simulink model "ABS_virtual_no_fliter_40_88"  (R2023a)
settings: Solver=VariableStepAuto  StartTime=0.0  StopTime=inf  FixedStep=0.001  RelTol=1e-3  EnableMultiTasking=on
PreLoadFcn:
  | SoftABS_params
libraries: CarMaker4SL x28, simulink x19, dspsigops x5
(part 2 of 3)

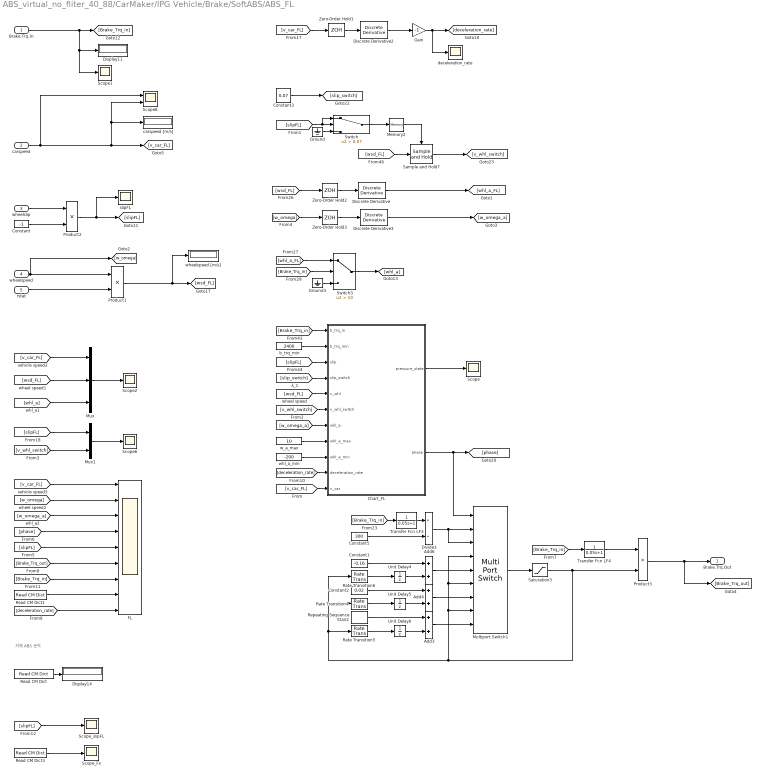
== system ABS_virtual_no_fliter_40_88/CarMaker/IPG Vehicle/Brake/SoftABS/ABS_FL ==
  note: 자체 ABS 로직
  Brake.Trq.In : Inport
  carspeed : Inport  Port=2
  wheelslip : Inport  Port=3
  wheelspeed : Inport  Port=4
  rstat : Inport  Port=5
  Add3 : Sum
  Add4 : Sum
  Add6 : Sum
  Chart_FL : Stateflow chart  TreatAsAtomicUnit=on
      settings: PortSchema="{\"entries\":[{\"content\":{\"sides\":[{\"content\":{\"connectorIds\":[\"In1\",\"In3\",\"In2\",\"In4\",\"In5\",\"In6\",\"In7\",\"In8\",\"In9\",\"In10\",\"In11\"]},\"type\":\"ConnectorPlacement.EquallySpacedRectSide\",\"uuid\":\"cdedcea2-93f8-4775-9e06-e6ef8db0f566\"},{\"content\":{\"connectorIds\":[\"Out1\",\"Out2\"],\"side\":\"RIGHT\"},\"type\":\"ConnectorPlacement.EquallySpacedRectSide\",\"uuid\":\"86cd5634-3296-4603-b9fe-1da91bf44691\"},{\"content\":{\"side\":\"TOP\"},\"type\":\"ConnectorPlacement.EquallySpacedRectSide\",\"uuid\":\"3d39226d-e82c-42be-bb61-abed7a445d69\"}]},\"type\":\"ConnectorPlacement.EquallySpacedConnector\",\"uuid\":\"e0869cc4-498e-4360-9359-f4884b7944df\"}],\"packageUris\":[\"http://schema.mathworks.com/mf0/Connector/R2020b\"],\"version\":\"1.0\"}"
  Constant : Constant  Value=-1
  Constant1 : Constant  Value=-0.16
  Constant2 : Constant  Value=0.02
  Constant3 : Constant  Value=0.07
  Constant5 : Constant  Value=300
  Discrete Derivative : simulink/Discrete/Discrete Derivative  gainval=1.0  ICPrevScaledInput=0.0  OutMin=[]  OutMax=[]  OutDataType=fixdt(1, 16)  OutScaling=2^-10  DoSatur=off
  Discrete Derivative2 : simulink/Discrete/Discrete Derivative  gainval=1.0  ICPrevScaledInput=0.0  OutMin=[]  OutMax=[]  OutDataType=fixdt(1, 16)  OutScaling=2^-10  DoSatur=off
  Discrete Derivative3 : simulink/Discrete/Discrete Derivative  gainval=1.0  ICPrevScaledInput=0.0  OutMin=[]  OutMax=[]  OutDataType=fixdt(1, 16)  OutScaling=2^-10  DoSatur=off
  Display11 : Display
  Display14 : Display
  Divide3 : Product  Inputs=*/
  FL : Scope  NumInputPorts=9
  Gain : Gain  Gain=-1
  Ground : Ground
  Ground3 : Ground
  Memory2 : Memory  InheritSampleTime=on
  Multiport Switch1 : MultiPortSwitch  DataPortOrder=Zero-based contiguous  Inputs=8  zeroidx=on  SaturateOnIntegerOverflow=off  InputSameDT=off
  Mux : Mux  Inputs=3
  Mux1 : Mux  Inputs=2
  Product1 : Product
  Product2 : Product
  Product3 : Product  InputSameDT=on  SaturateOnIntegerOverflow=on  OutDataTypeStr=Inherit: Same as first input
  Rate Transition4 : RateTransition  OutPortSampleTime=0.001
  Rate Transition5 : RateTransition  OutPortSampleTime=0.001
  Rate Transition6 : RateTransition  OutPortSampleTime=0.001
  Read CM Dict : CarMaker4SL/Read CM Dict  xname=DM.Long.StepDist  xsync=off  xstime=Continuous
  Read CM Dict1 : CarMaker4SL/Read CM Dict  xname=Car.FxFL  xsync=off  xstime=Continuous
  Read CM Dict3 : CarMaker4SL/Read CM Dict  xname=Car.FxFL  xsync=off  xstime=Continuous
  Repeating Sequence Stair2 : simulink/Sources/Repeating Sequence Stair  OutValues=[0.02 0].'  tsamp=0.001  OutMin=[]  OutMax=[]  OutDataTypeStr=double  OutputDataTypeScalingMode=double  OutDataType=fixdt(0,8)  ConRadixGroup=Best Precision: Vector-wise  OutScaling=2^-12
  Sample and Hold7 : dspsigops/Sample and Hold  trig=Rising edge  initCond=0  latchinput=off
  Saturation3 : Saturate  UpperLimit=1  LowerLimit=0
  Scope{,1..2,6} (4 alike) : Scope
  Scope8 : Scope  NumInputPorts=2
  Scope_Fx : Scope
  Scope_slipFL : Scope
  Switch : Switch  Criteria=u2 > Threshold  Threshold=0.07  SaturateOnIntegerOverflow=off  InputSameDT=off
  Switch3 : Switch  Criteria=u2 > Threshold  Threshold=10  SaturateOnIntegerOverflow=off  InputSameDT=off
  Transfer Fcn LF3 : TransferFcn  Denominator=[0.05 1]
  Transfer Fcn LF4 : TransferFcn  Denominator=[0.05 1]
  Unit Delay4 : UnitDelay  SampleTime=0.001  HasFrameUpgradeWarning=on
  Unit Delay5 : UnitDelay  SampleTime=0.001  HasFrameUpgradeWarning=on
  Unit Delay6 : UnitDelay  SampleTime=0.001  HasFrameUpgradeWarning=on
  Zero-Order Hold1 : ZeroOrderHold  SampleTime=0.001
  Zero-Order Hold2 : ZeroOrderHold  SampleTime=0.001
  Zero-Order Hold3 : ZeroOrderHold  SampleTime=0.001
  b_trq_min : Constant  Value=2400
  carspeed [m/s] : Display
  deceleration_rate : Scope
  slipFL : Scope
  w_a_max : Constant  Value=10
  wheelspeed [m/s] : Display
  whl_a_min : Constant  Value=-200
  Brake.Trq.Out : Outport  VectorParamsAs1DForOutWhenUnconnected=off
  wires:
  [wsd_FL] -> Zero-Order Hold2/1
  rstat/1 -> Product1/2
  Brake.Trq.In/1 -> Scope1/1, Display11/1, [Brake_Trq_in]
  Read CM Dict/1 -> Display14/1
  wheelslip/1 -> Product2/1
  Product2/1 -> slipFL/1, [slipFL]
  Constant/1 -> Product2/2
  carspeed/1 -> [v_car_FL], Scope8/2, carspeed [m/s]/1, Scope8/1
  [Brake_Trq_in] -> Switch3/2
  Ground3/1 -> Switch3/3
  Switch3/1 -> [whl_a]
  [whl_a_FL] -> Switch3/1
  [Brake_Trq_in] -> Chart_FL/1(b_trq_in)
  b_trq_min/1 -> Chart_FL/3(b_trq_min)
  [slipFL] -> Chart_FL/2(slip)
  Chart_FL/2(phase) -> [phase], Multiport Switch1/1
  Chart_FL/1(pressure_state) -> Scope/1
  [slipFL] -> Switch/1, Switch/2
  Constant3/1 -> [slip_switch]
  Switch/1 -> Memory2/1
  [wsd_FL] -> Sample and Hold7/1
  Sample and Hold7/1 -> [v_whl_switch]
  [slip_switch] -> Chart_FL/4(slip_switch)
  [w_omega_a] -> Chart_FL/7(whl_a)
  whl_a_min/1 -> Chart_FL/9(whl_a_min)
  w_a_max/1 -> Chart_FL/8(whl_a_max)
  [wsd_FL] -> Chart_FL/5(v_whl)
  Ground/1 -> Switch/3
  Memory2/1 -> Sample and Hold7/Trigger
  [v_car_FL] -> Mux/1
  [wsd_FL] -> Mux/2
  [whl_a] -> Mux/3
  Mux/1 -> Scope2/1
  [slipFL] -> Mux1/1
  [v_whl_switch] -> Mux1/2
  Mux1/1 -> Scope6/1
  [w_omega] -> FL/2
  [v_car_FL] -> FL/1
  [w_omega_a] -> FL/3
  [phase] -> FL/4
  [slipFL] -> FL/5
  [Brake_Trq_out] -> FL/6
  [Brake_Trq_in] -> FL/7
  Read CM Dict1/1 -> FL/8
  Discrete Derivative2/1 -> Gain/1
  Gain/1 -> deceleration_rate/1, [deceleration_rate]
  [v_car_FL] -> Chart_FL/11(v_car)
  [v_car_FL] -> Zero-Order Hold1/1
  [v_whl_switch] -> Chart_FL/6(v_whl_switch)
  [w_omega] -> Zero-Order Hold3/1
  wheelspeed/1 -> [w_omega], Product1/1
  Discrete Derivative/1 -> [whl_a_FL]
  Product1/1 -> [wsd_FL], wheelspeed [m/s]/1
  Zero-Order Hold1/1 -> Discrete Derivative2/1
  Zero-Order Hold2/1 -> Discrete Derivative/1
  Zero-Order Hold3/1 -> Discrete Derivative3/1
  Rate Transition4/1 -> Unit Delay5/1
  Unit Delay5/1 -> Add4/2
  Add4/1 -> Multiport Switch1/7
  Transfer Fcn LF4/1 -> Product3/1
  Repeating Sequence Stair2/1 -> Add3/1
  [Brake_Trq_in] -> Transfer Fcn LF3/1
  Add3/1 -> Multiport Switch1/9
  Saturation3/1 -> Multiport Switch1/8, Multiport Switch1/6, Multiport Switch1/4, Rate Transition5/1, Rate Transition4/1, Rate Transition6/1, Product3/2
  Multiport Switch1/1 -> Saturation3/1
  [Brake_Trq_in] -> Transfer Fcn LF4/1
  Divide3/1 -> Multiport Switch1/3, Multiport Switch1/2
  Product3/1 -> Brake.Trq.Out/1, [Brake_Trq_out]
  Unit Delay4/1 -> Add6/2
  Constant2/1 -> Add4/1
  Transfer Fcn LF3/1 -> Divide3/1
  Rate Transition5/1 -> Unit Delay6/1
  Constant1/1 -> Add6/1
  Unit Delay6/1 -> Add3/2
  Rate Transition6/1 -> Unit Delay4/1
  Constant5/1 -> Divide3/2
  Add6/1 -> Multiport Switch1/5
  Discrete Derivative3/1 -> [w_omega_a]
  [deceleration_rate] -> FL/9
  [deceleration_rate] -> Chart_FL/10(deceleration_rate)
  Read CM Dict3/1 -> Scope_Fx/1
  [slipFL] -> Scope_slipFL/1

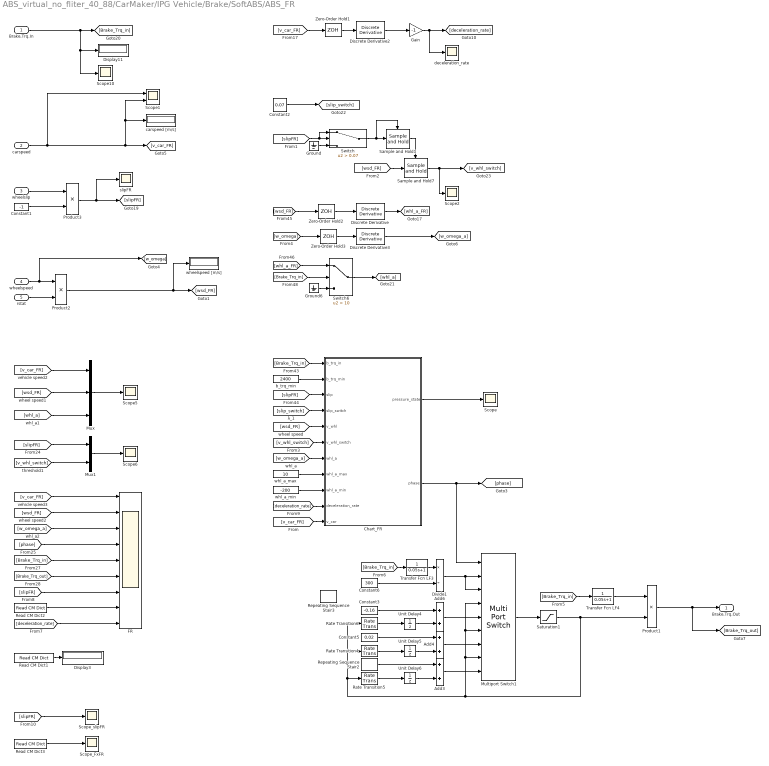
== system ABS_virtual_no_fliter_40_88/CarMaker/IPG Vehicle/Brake/SoftABS/ABS_FR ==
  Brake.Trq.In : Inport
  carspeed : Inport  Port=2
  wheelslip : Inport  Port=3
  wheelspeed : Inport  Port=4
  rstat : Inport  Port=5
  Add3 : Sum
  Add4 : Sum
  Add6 : Sum
  Chart_FR : Stateflow chart  TreatAsAtomicUnit=on
      settings: PortSchema="{\"entries\":[{\"content\":{\"sides\":[{\"content\":{\"connectorIds\":[\"In1\",\"In3\",\"In2\",\"In4\",\"In5\",\"In6\",\"In7\",\"In8\",\"In9\",\"In10\",\"In11\"]},\"type\":\"ConnectorPlacement.EquallySpacedRectSide\",\"uuid\":\"cdedcea2-93f8-4775-9e06-e6ef8db0f566\"},{\"content\":{\"connectorIds\":[\"Out1\",\"Out2\"],\"side\":\"RIGHT\"},\"type\":\"ConnectorPlacement.EquallySpacedRectSide\",\"uuid\":\"86cd5634-3296-4603-b9fe-1da91bf44691\"},{\"content\":{\"side\":\"TOP\"},\"type\":\"ConnectorPlacement.EquallySpacedRectSide\",\"uuid\":\"3d39226d-e82c-42be-bb61-abed7a445d69\"}]},\"type\":\"ConnectorPlacement.EquallySpacedConnector\",\"uuid\":\"e0869cc4-498e-4360-9359-f4884b7944df\"}],\"packageUris\":[\"http://schema.mathworks.com/mf0/Connector/R2020b\"],\"version\":\"1.0\"}"
  Constant1 : Constant  Value=-1
  Constant2 : Constant  Value=0.07
  Constant3 : Constant  Value=-0.16
  Constant5 : Constant  Value=0.02
  Constant6 : Constant  Value=300
  Discrete Derivative : simulink/Discrete/Discrete Derivative  gainval=1.0  ICPrevScaledInput=0.0  OutMin=[]  OutMax=[]  OutDataType=fixdt(1, 16)  OutScaling=2^-10  DoSatur=off
  Discrete Derivative2 : simulink/Discrete/Discrete Derivative  gainval=1.0  ICPrevScaledInput=0.0  OutMin=[]  OutMax=[]  OutDataType=fixdt(1, 16)  OutScaling=2^-10  DoSatur=off
  Discrete Derivative3 : simulink/Discrete/Discrete Derivative  gainval=1.0  ICPrevScaledInput=0.0  OutMin=[]  OutMax=[]  OutDataType=fixdt(1, 16)  OutScaling=2^-10  DoSatur=off
  Display11 : Display
  Display3 : Display
  Divide1 : Product  Inputs=*/
  FR : Scope  NumInputPorts=9
  Gain : Gain  Gain=-1
  Ground : Ground
  Ground6 : Ground
  Multiport Switch1 : MultiPortSwitch  DataPortOrder=Zero-based contiguous  Inputs=8  zeroidx=on  SaturateOnIntegerOverflow=off  InputSameDT=off
  Mux : Mux  Inputs=3
  Mux1 : Mux  Inputs=2
  Product1 : Product  InputSameDT=on  SaturateOnIntegerOverflow=on  OutDataTypeStr=Inherit: Same as first input
  Product2 : Product
  Product3 : Product
  Rate Transition4 : RateTransition  OutPortSampleTime=0.001
  Rate Transition5 : RateTransition  OutPortSampleTime=0.001
  Rate Transition6 : RateTransition  OutPortSampleTime=0.001
  Read CM Dict1 : CarMaker4SL/Read CM Dict  xname=DM.Long.StepDist  xsync=off  xstime=Continuous
  Read CM Dict2 : CarMaker4SL/Read CM Dict  xname=Car.FxFR  xsync=off  xstime=Continuous
  Read CM Dict3 : CarMaker4SL/Read CM Dict  xname=Car.FxFR  xsync=off  xstime=Continuous
  Repeating Sequence Stair2 : simulink/Sources/Repeating Sequence Stair  OutValues=[0.02 0].'  tsamp=0.001  OutMin=[]  OutMax=[]  OutDataTypeStr=double  OutputDataTypeScalingMode=double  OutDataType=fixdt(0,8)  ConRadixGroup=Best Precision: Vector-wise  OutScaling=2^-12
  Repeating Sequence Stair3 : simulink/Sources/Repeating Sequence Stair  OutValues=[-0.16 0].'  tsamp=0.001  OutMin=[]  OutMax=[]  OutDataTypeStr=double  OutputDataTypeScalingMode=double  OutDataType=fixdt(0,8)  ConRadixGroup=Best Precision: Vector-wise  OutScaling=2^-12
  Sample and Hold1 : dspsigops/Sample and Hold  trig=Rising edge  initCond=0  latchinput=off
  Sample and Hold7 : dspsigops/Sample and Hold  trig=Rising edge  initCond=0  latchinput=off
  Saturation1 : Saturate  UpperLimit=1  LowerLimit=0
  Scope{,2,5..6,10} (5 alike) : Scope
  Scope1 : Scope  NumInputPorts=2
  Scope_FxFR : Scope
  Scope_slipFR : Scope
  Switch : Switch  Criteria=u2 > Threshold  Threshold=0.07  SaturateOnIntegerOverflow=off  InputSameDT=off
  Switch6 : Switch  Criteria=u2 > Threshold  Threshold=10  SaturateOnIntegerOverflow=off  InputSameDT=off
  Transfer Fcn LF3 : TransferFcn  Denominator=[0.05 1]
  Transfer Fcn LF4 : TransferFcn  Denominator=[0.05 1]
  Unit Delay4 : UnitDelay  SampleTime=0.001  HasFrameUpgradeWarning=on
  Unit Delay5 : UnitDelay  SampleTime=0.001  HasFrameUpgradeWarning=on
  Unit Delay6 : UnitDelay  SampleTime=0.001  HasFrameUpgradeWarning=on
  Zero-Order Hold1 : ZeroOrderHold  SampleTime=0.001
  Zero-Order Hold2 : ZeroOrderHold  SampleTime=0.001
  Zero-Order Hold3 : ZeroOrderHold  SampleTime=0.001
  b_trq_min : Constant  Value=2400
  carspeed [m/s] : Display
  deceleration_rate : Scope
  slipFR : Scope
  wheelspeed [m/s] : Display
  whl_a_max : Constant  Value=10
  whl_a_min : Constant  Value=-200
  Brake.Trq.Out : Outport  VectorParamsAs1DForOutWhenUnconnected=off
  wires:
  Switch6/1 -> [whl_a]
  Read CM Dict1/1 -> Display3/1
  Ground6/1 -> Switch6/3
  [Brake_Trq_in] -> Switch6/2
  [whl_a_FR] -> Switch6/1
  wheelslip/1 -> Product3/1
  Constant1/1 -> Product3/2
  Product3/1 -> slipFR/1, [slipFR]
  rstat/1 -> Product2/2
  Discrete Derivative/1 -> [whl_a_FR]
  Brake.Trq.In/1 -> Scope10/1, Display11/1, [Brake_Trq_in]
  [wsd_FR] -> Zero-Order Hold2/1
  carspeed/1 -> Scope1/2, carspeed [m/s]/1, [v_car_FR], Scope1/1
  Constant2/1 -> [slip_switch]
  Chart_FR/1(pressure_state) -> Scope/1
  Chart_FR/2(phase) -> [phase], Multiport Switch1/1
  [whl_a] -> Mux/3
  [slipFR] -> FR/7
  [wsd_FR] -> Mux/2
  Mux/1 -> Scope5/1
  [v_whl_switch] -> Mux1/2
  [slipFR] -> Mux1/1
  [v_car_FR] -> FR/1
  [Brake_Trq_in] -> FR/5
  [w_omega_a] -> FR/3
  [Brake_Trq_out] -> FR/6
  [v_car_FR] -> Mux/1
  [phase] -> FR/4
  [wsd_FR] -> FR/2
  Mux1/1 -> Scope6/1
  Read CM Dict2/1 -> FR/8
  Product2/1 -> [wsd_FR], wheelspeed [m/s]/1
  Discrete Derivative2/1 -> Gain/1
  [v_car_FR] -> Zero-Order Hold1/1
  Gain/1 -> deceleration_rate/1, [deceleration_rate]
  [v_whl_switch] -> Chart_FR/6(v_whl_switch)
  b_trq_min/1 -> Chart_FR/3(b_trq_min)
  [v_car_FR] -> Chart_FR/11(v_car)
  whl_a_max/1 -> Chart_FR/8(whl_a_max)
  [w_omega_a] -> Chart_FR/7(whl_a)
  [slipFR] -> Chart_FR/2(slip)
  [wsd_FR] -> Chart_FR/5(v_whl)
  [Brake_Trq_in] -> Chart_FR/1(b_trq_in)
  whl_a_min/1 -> Chart_FR/9(whl_a_min)
  [slip_switch] -> Chart_FR/4(slip_switch)
  Switch/1 -> Sample and Hold1/1, Sample and Hold1/Trigger
  Ground/1 -> Switch/3
  [wsd_FR] -> Sample and Hold7/1
  [slipFR] -> Switch/1, Switch/2
  Sample and Hold7/1 -> Scope2/1, [v_whl_switch]
  [w_omega] -> Zero-Order Hold3/1
  wheelspeed/1 -> [w_omega], Product2/1
  Sample and Hold1/1 -> Sample and Hold7/Trigger
  Zero-Order Hold1/1 -> Discrete Derivative2/1
  Zero-Order Hold2/1 -> Discrete Derivative/1
  Zero-Order Hold3/1 -> Discrete Derivative3/1
  Rate Transition4/1 -> Unit Delay5/1
  Unit Delay5/1 -> Add4/2
  Add4/1 -> Multiport Switch1/7
  Transfer Fcn LF4/1 -> Product1/1
  Repeating Sequence Stair2/1 -> Add3/1
  [Brake_Trq_in] -> Transfer Fcn LF3/1
  Add3/1 -> Multiport Switch1/9
  Saturation1/1 -> Multiport Switch1/8, Multiport Switch1/6, Multiport Switch1/4, Rate Transition6/1, Rate Transition4/1, Rate Transition5/1, Product1/2
  Multiport Switch1/1 -> Saturation1/1
  [Brake_Trq_in] -> Transfer Fcn LF4/1
  Divide1/1 -> Multiport Switch1/3, Multiport Switch1/2
  Product1/1 -> Brake.Trq.Out/1, [Brake_Trq_out]
  Unit Delay4/1 -> Add6/2
  Constant5/1 -> Add4/1
  Transfer Fcn LF3/1 -> Divide1/1
  Rate Transition5/1 -> Unit Delay6/1
  Constant3/1 -> Add6/1
  Unit Delay6/1 -> Add3/2
  Rate Transition6/1 -> Unit Delay4/1
  Constant6/1 -> Divide1/2
  Add6/1 -> Multiport Switch1/5
  Discrete Derivative3/1 -> [w_omega_a]
  [deceleration_rate] -> FR/9
  [deceleration_rate] -> Chart_FR/10(deceleration_rate)
  Read CM Dict3/1 -> Scope_FxFR/1
  [slipFR] -> Scope_slipFR/1

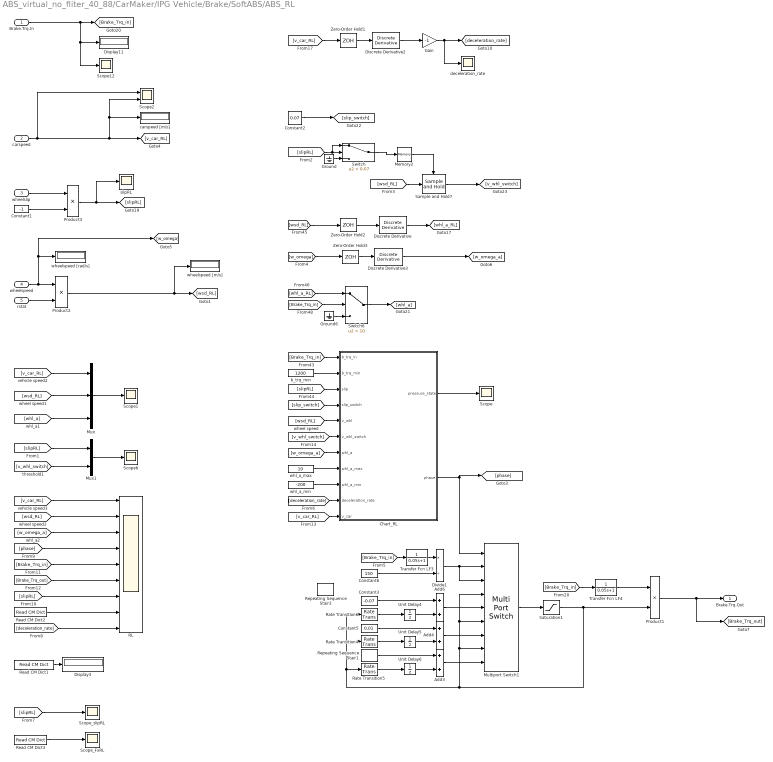
== system ABS_virtual_no_fliter_40_88/CarMaker/IPG Vehicle/Brake/SoftABS/ABS_RL ==
  Brake.Trq.In : Inport
  carspeed : Inport  Port=2
  wheelslip : Inport  Port=3
  wheelspeed : Inport  Port=4
  rstat : Inport  Port=5
  Add3 : Sum
  Add4 : Sum
  Add6 : Sum
  Chart_RL : Stateflow chart  TreatAsAtomicUnit=on
      settings: PortSchema="{\"entries\":[{\"content\":{\"sides\":[{\"content\":{\"connectorIds\":[\"In1\",\"In3\",\"In2\",\"In4\",\"In5\",\"In6\",\"In7\",\"In8\",\"In9\",\"In10\",\"In11\"]},\"type\":\"ConnectorPlacement.EquallySpacedRectSide\",\"uuid\":\"cdedcea2-93f8-4775-9e06-e6ef8db0f566\"},{\"content\":{\"connectorIds\":[\"Out1\",\"Out2\"],\"side\":\"RIGHT\"},\"type\":\"ConnectorPlacement.EquallySpacedRectSide\",\"uuid\":\"86cd5634-3296-4603-b9fe-1da91bf44691\"},{\"content\":{\"side\":\"TOP\"},\"type\":\"ConnectorPlacement.EquallySpacedRectSide\",\"uuid\":\"3d39226d-e82c-42be-bb61-abed7a445d69\"}]},\"type\":\"ConnectorPlacement.EquallySpacedConnector\",\"uuid\":\"e0869cc4-498e-4360-9359-f4884b7944df\"}],\"packageUris\":[\"http://schema.mathworks.com/mf0/Connector/R2020b\"],\"version\":\"1.0\"}"
  Constant1 : Constant  Value=-1
  Constant2 : Constant  Value=0.07
  Constant3 : Constant  Value=-0.07
  Constant5 : Constant  Value=0.01
  Constant6 : Constant  Value=150
  Discrete Derivative : simulink/Discrete/Discrete Derivative  gainval=1.0  ICPrevScaledInput=0.0  OutMin=[]  OutMax=[]  OutDataType=fixdt(1, 16)  OutScaling=2^-10  DoSatur=off
  Discrete Derivative2 : simulink/Discrete/Discrete Derivative  gainval=1.0  ICPrevScaledInput=0.0  OutMin=[]  OutMax=[]  OutDataType=fixdt(1, 16)  OutScaling=2^-10  DoSatur=off
  Discrete Derivative3 : simulink/Discrete/Discrete Derivative  gainval=1.0  ICPrevScaledInput=0.0  OutMin=[]  OutMax=[]  OutDataType=fixdt(1, 16)  OutScaling=2^-10  DoSatur=off
  Display11 : Display
  Display3 : Display
  Divide1 : Product  Inputs=*/
  Gain : Gain  Gain=-1
  Ground : Ground
  Ground6 : Ground
  Memory2 : Memory  InheritSampleTime=on
  Multiport Switch1 : MultiPortSwitch  DataPortOrder=Zero-based contiguous  Inputs=8  zeroidx=on  SaturateOnIntegerOverflow=off  InputSameDT=off
  Mux : Mux  Inputs=3
  Mux1 : Mux  Inputs=2
  Product1 : Product  InputSameDT=on  SaturateOnIntegerOverflow=on  OutDataTypeStr=Inherit: Same as first input
  Product2 : Product
  Product3 : Product
  RL : Scope  NumInputPorts=9
  Rate Transition4 : RateTransition  OutPortSampleTime=0.001
  Rate Transition5 : RateTransition  OutPortSampleTime=0.001
  Rate Transition6 : RateTransition  OutPortSampleTime=0.001
  Read CM Dict1 : CarMaker4SL/Read CM Dict  xname=DM.Long.StepDist  xsync=off  xstime=Continuous
  Read CM Dict2 : CarMaker4SL/Read CM Dict  xname=Car.FxRL  xsync=off  xstime=Continuous
  Read CM Dict3 : CarMaker4SL/Read CM Dict  xname=Car.FxRL  xsync=off  xstime=Continuous
  Repeating Sequence Stair1 : simulink/Sources/Repeating Sequence Stair  OutValues=[0.07 0].'  tsamp=0.001  OutMin=[]  OutMax=[]  OutDataTypeStr=double  OutputDataTypeScalingMode=double  OutDataType=fixdt(0,8)  ConRadixGroup=Best Precision: Vector-wise  OutScaling=2^-12
  Repeating Sequence Stair3 : simulink/Sources/Repeating Sequence Stair  OutValues=[-0.07 0].'  tsamp=0.001  OutMin=[]  OutMax=[]  OutDataTypeStr=double  OutputDataTypeScalingMode=double  OutDataType=fixdt(0,8)  ConRadixGroup=Best Precision: Vector-wise  OutScaling=2^-12
  Sample and Hold7 : dspsigops/Sample and Hold  trig=Rising edge  initCond=0  latchinput=off
  Saturation1 : Saturate  UpperLimit=1  LowerLimit=0
  Scope{,1,6,12} (4 alike) : Scope
  Scope2 : Scope  NumInputPorts=2
  Scope_FxRL : Scope
  Scope_slipRL : Scope
  Switch : Switch  Criteria=u2 > Threshold  Threshold=0.07  SaturateOnIntegerOverflow=off  InputSameDT=off
  Switch6 : Switch  Criteria=u2 > Threshold  Threshold=10  SaturateOnIntegerOverflow=off  InputSameDT=off
  Transfer Fcn LF3 : TransferFcn  Denominator=[0.05 1]
  Transfer Fcn LF4 : TransferFcn  Denominator=[0.05 1]
  Unit Delay4 : UnitDelay  SampleTime=0.001  HasFrameUpgradeWarning=on
  Unit Delay5 : UnitDelay  SampleTime=0.001  HasFrameUpgradeWarning=on
  Unit Delay6 : UnitDelay  SampleTime=0.001  HasFrameUpgradeWarning=on
  Zero-Order Hold1 : ZeroOrderHold  SampleTime=0.001
  Zero-Order Hold2 : ZeroOrderHold  SampleTime=0.001
  Zero-Order Hold3 : ZeroOrderHold  SampleTime=0.001
  b_trq_min : Constant  Value=1200
  carspeed [m/s] : Display
  deceleration_rate : Scope
  slipRL : Scope
  wheelspeed [m/s] : Display
  wheelspeed [rad/s] : Display
  whl_a_max : Constant  Value=10
  whl_a_min : Constant  Value=-200
  Brake.Trq.Out : Outport  VectorParamsAs1DForOutWhenUnconnected=off
  wires:
  Switch6/1 -> [whl_a]
  Read CM Dict1/1 -> Display3/1
  Ground6/1 -> Switch6/3
  [Brake_Trq_in] -> Switch6/2
  [whl_a_RL] -> Switch6/1
  wheelslip/1 -> Product3/1
  Constant1/1 -> Product3/2
  Product3/1 -> slipRL/1, [slipRL]
  rstat/1 -> Product2/2
  Discrete Derivative/1 -> [whl_a_RL]
  Brake.Trq.In/1 -> Scope12/1, Display11/1, [Brake_Trq_in]
  [wsd_RL] -> Zero-Order Hold2/1
  carspeed/1 -> [v_car_RL], Scope2/2, carspeed [m/s]/1, Scope2/1
  Chart_RL/2(phase) -> [phase], Multiport Switch1/1
  Constant2/1 -> [slip_switch]
  Chart_RL/1(pressure_state) -> Scope/1
  [whl_a] -> Mux/3
  [slipRL] -> RL/7
  [wsd_RL] -> Mux/2
  Mux/1 -> Scope1/1
  [v_whl_switch] -> Mux1/2
  [slipRL] -> Mux1/1
  [v_car_RL] -> RL/1
  [Brake_Trq_in] -> RL/5
  [w_omega_a] -> RL/3
  [Brake_Trq_out] -> RL/6
  [v_car_RL] -> Mux/1
  [phase] -> RL/4
  [wsd_RL] -> RL/2
  Mux1/1 -> Scope6/1
  Read CM Dict2/1 -> RL/8
  Product2/1 -> [wsd_RL], wheelspeed [m/s]/1
  Discrete Derivative2/1 -> Gain/1
  [v_car_RL] -> Zero-Order Hold1/1
  Gain/1 -> deceleration_rate/1, [deceleration_rate]
  Switch/1 -> Memory2/1
  Memory2/1 -> Sample and Hold7/Trigger
  Ground/1 -> Switch/3
  [wsd_RL] -> Sample and Hold7/1
  [slipRL] -> Switch/1, Switch/2
  Sample and Hold7/1 -> [v_whl_switch]
  [v_whl_switch] -> Chart_RL/6(v_whl_switch)
  b_trq_min/1 -> Chart_RL/3(b_trq_min)
  [v_car_RL] -> Chart_RL/11(v_car)
  whl_a_max/1 -> Chart_RL/8(whl_a_max)
  [w_omega_a] -> Chart_RL/7(whl_a)
  [slipRL] -> Chart_RL/2(slip)
  [wsd_RL] -> Chart_RL/5(v_whl)
  [Brake_Trq_in] -> Chart_RL/1(b_trq_in)
  whl_a_min/1 -> Chart_RL/9(whl_a_min)
  [slip_switch] -> Chart_RL/4(slip_switch)
  [w_omega] -> Zero-Order Hold3/1
  wheelspeed/1 -> [w_omega], wheelspeed [rad/s]/1, Product2/1
  Zero-Order Hold1/1 -> Discrete Derivative2/1
  Zero-Order Hold2/1 -> Discrete Derivative/1
  Zero-Order Hold3/1 -> Discrete Derivative3/1
  Rate Transition4/1 -> Unit Delay5/1
  Unit Delay5/1 -> Add4/2
  Add4/1 -> Multiport Switch1/7
  Transfer Fcn LF4/1 -> Product1/1
  Repeating Sequence Stair1/1 -> Add3/1
  [Brake_Trq_in] -> Transfer Fcn LF3/1
  Add3/1 -> Multiport Switch1/9
  Saturation1/1 -> Multiport Switch1/8, Multiport Switch1/6, Multiport Switch1/4, Rate Transition6/1, Rate Transition4/1, Rate Transition5/1, Product1/2
  Multiport Switch1/1 -> Saturation1/1
  [Brake_Trq_in] -> Transfer Fcn LF4/1
  Divide1/1 -> Multiport Switch1/3, Multiport Switch1/2
  Product1/1 -> Brake.Trq.Out/1, [Brake_Trq_out]
  Unit Delay4/1 -> Add6/2
  Constant5/1 -> Add4/1
  Transfer Fcn LF3/1 -> Divide1/1
  Rate Transition5/1 -> Unit Delay6/1
  Constant3/1 -> Add6/1
  Unit Delay6/1 -> Add3/2
  Rate Transition6/1 -> Unit Delay4/1
  Constant6/1 -> Divide1/2
  Add6/1 -> Multiport Switch1/5
  Discrete Derivative3/1 -> [w_omega_a]
  [deceleration_rate] -> RL/9
  [deceleration_rate] -> Chart_RL/10(deceleration_rate)
  Read CM Dict3/1 -> Scope_FxRL/1
  [slipRL] -> Scope_slipRL/1

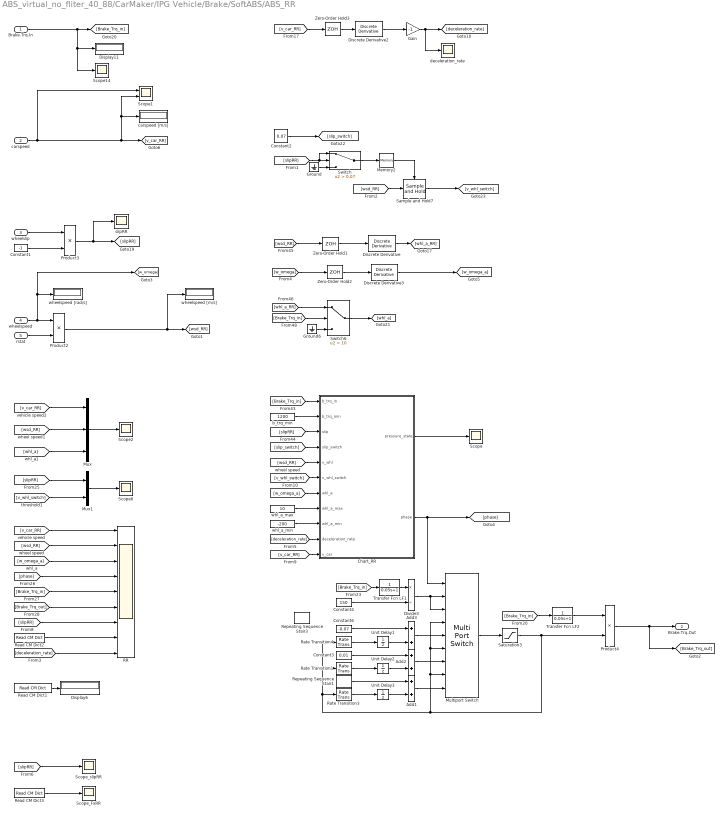
== system ABS_virtual_no_fliter_40_88/CarMaker/IPG Vehicle/Brake/SoftABS/ABS_RR ==
  Brake.Trq.In : Inport
  carspeed : Inport  Port=2
  wheelslip : Inport  Port=3
  wheelspeed : Inport  Port=4
  rstat : Inport  Port=5
  Add1 : Sum
  Add2 : Sum
  Add3 : Sum
  Chart_RR : Stateflow chart  TreatAsAtomicUnit=on
      settings: PortSchema="{\"entries\":[{\"content\":{\"sides\":[{\"content\":{\"connectorIds\":[\"In1\",\"In3\",\"In2\",\"In4\",\"In5\",\"In6\",\"In7\",\"In8\",\"In9\",\"In10\",\"In11\"]},\"type\":\"ConnectorPlacement.EquallySpacedRectSide\",\"uuid\":\"cdedcea2-93f8-4775-9e06-e6ef8db0f566\"},{\"content\":{\"connectorIds\":[\"Out1\",\"Out2\"],\"side\":\"RIGHT\"},\"type\":\"ConnectorPlacement.EquallySpacedRectSide\",\"uuid\":\"86cd5634-3296-4603-b9fe-1da91bf44691\"},{\"content\":{\"side\":\"TOP\"},\"type\":\"ConnectorPlacement.EquallySpacedRectSide\",\"uuid\":\"3d39226d-e82c-42be-bb61-abed7a445d69\"}]},\"type\":\"ConnectorPlacement.EquallySpacedConnector\",\"uuid\":\"e0869cc4-498e-4360-9359-f4884b7944df\"}],\"packageUris\":[\"http://schema.mathworks.com/mf0/Connector/R2020b\"],\"version\":\"1.0\"}"
  Constant1 : Constant  Value=-1
  Constant2 : Constant  Value=0.07
  Constant3 : Constant  Value=0.01
  Constant4 : Constant  Value=150
  Constant6 : Constant  Value=-0.07
  Discrete Derivative : simulink/Discrete/Discrete Derivative  gainval=1.0  ICPrevScaledInput=0.0  OutMin=[]  OutMax=[]  OutDataType=fixdt(1, 16)  OutScaling=2^-10  DoSatur=off
  Discrete Derivative2 : simulink/Discrete/Discrete Derivative  gainval=1.0  ICPrevScaledInput=0.0  OutMin=[]  OutMax=[]  OutDataType=fixdt(1, 16)  OutScaling=2^-10  DoSatur=off
  Discrete Derivative3 : simulink/Discrete/Discrete Derivative  gainval=1.0  ICPrevScaledInput=0.0  OutMin=[]  OutMax=[]  OutDataType=fixdt(1, 16)  OutScaling=2^-10  DoSatur=off
  Display11 : Display
  Display6 : Display
  Divide3 : Product  Inputs=*/
  Gain : Gain  Gain=-1
  Ground : Ground
  Ground6 : Ground
  Memory2 : Memory  InheritSampleTime=on
  Multiport Switch : MultiPortSwitch  DataPortOrder=Zero-based contiguous  Inputs=8  zeroidx=on  SaturateOnIntegerOverflow=off  InputSameDT=off
  Mux : Mux  Inputs=3
  Mux1 : Mux  Inputs=2
  Product2 : Product
  Product3 : Product
  Product4 : Product  InputSameDT=on  SaturateOnIntegerOverflow=on  OutDataTypeStr=Inherit: Same as first input
  RR : Scope  NumInputPorts=9
  Rate Transition1 : RateTransition  OutPortSampleTime=0.001
  Rate Transition3 : RateTransition  OutPortSampleTime=0.001
  Rate Transition4 : RateTransition  OutPortSampleTime=0.001
  Read CM Dict1 : CarMaker4SL/Read CM Dict  xname=DM.Long.StepDist  xsync=off  xstime=Continuous
  Read CM Dict2 : CarMaker4SL/Read CM Dict  xname=Car.FxRR  xsync=off  xstime=Continuous
  Read CM Dict3 : CarMaker4SL/Read CM Dict  xname=Car.FxRR  xsync=off  xstime=Continuous
  Repeating Sequence Stair1 : simulink/Sources/Repeating Sequence Stair  OutValues=[0.07 0].'  tsamp=0.001  OutMin=[]  OutMax=[]  OutDataTypeStr=double  OutputDataTypeScalingMode=double  OutDataType=fixdt(0,8)  ConRadixGroup=Best Precision: Vector-wise  OutScaling=2^-12
  Repeating Sequence Stair3 : simulink/Sources/Repeating Sequence Stair  OutValues=[-0.07 0].'  tsamp=0.001  OutMin=[]  OutMax=[]  OutDataTypeStr=double  OutputDataTypeScalingMode=double  OutDataType=fixdt(0,8)  ConRadixGroup=Best Precision: Vector-wise  OutScaling=2^-12
  Sample and Hold7 : dspsigops/Sample and Hold  trig=Rising edge  initCond=0  latchinput=off
  Saturation3 : Saturate  UpperLimit=1  LowerLimit=0
  Scope{,2,6,14} (4 alike) : Scope
  Scope1 : Scope  NumInputPorts=2
  Scope_FxRR : Scope
  Scope_slipRR : Scope
  Switch : Switch  Criteria=u2 > Threshold  Threshold=0.07  SaturateOnIntegerOverflow=off  InputSameDT=off
  Switch6 : Switch  Criteria=u2 > Threshold  Threshold=10  SaturateOnIntegerOverflow=off  InputSameDT=off
  Transfer Fcn LF1 : TransferFcn  Denominator=[0.05 1]
  Transfer Fcn LF2 : TransferFcn  Denominator=[0.05 1]
  Unit Delay1 : UnitDelay  SampleTime=0.001  HasFrameUpgradeWarning=on
  Unit Delay2 : UnitDelay  SampleTime=0.001  HasFrameUpgradeWarning=on
  Unit Delay3 : UnitDelay  SampleTime=0.001  HasFrameUpgradeWarning=on
  Zero-Order Hold1 : ZeroOrderHold  SampleTime=0.001
  Zero-Order Hold2 : ZeroOrderHold  SampleTime=0.001
  Zero-Order Hold3 : ZeroOrderHold  SampleTime=0.001
  b_trq_min : Constant  Value=1200
  carspeed [m/s] : Display
  deceleration_rate : Scope
  slipRR : Scope
  wheelspeed [m/s] : Display
  wheelspeed [rad/s] : Display
  whl_a_max : Constant  Value=10
  whl_a_min : Constant  Value=-200
  Brake.Trq.Out : Outport  VectorParamsAs1DForOutWhenUnconnected=off
  wires:
  Constant1/1 -> Product3/2
  wheelslip/1 -> Product3/1
  [whl_a_RR] -> Switch6/1
  Ground6/1 -> Switch6/3
  [Brake_Trq_in] -> Switch6/2
  Switch6/1 -> [whl_a]
  [wsd_RR] -> Zero-Order Hold1/1
  Brake.Trq.In/1 -> Scope14/1, Display11/1, [Brake_Trq_in]
  Read CM Dict1/1 -> Display6/1
  rstat/1 -> Product2/2
  Product3/1 -> slipRR/1, [slipRR]
  Discrete Derivative/1 -> [whl_a_RR]
  Product2/1 -> [wsd_RR], wheelspeed [m/s]/1
  Chart_RR/2(phase) -> [phase], Multiport Switch/1
  Constant2/1 -> [slip_switch]
  carspeed/1 -> [v_car_RR], Scope1/2, carspeed [m/s]/1, Scope1/1
  Multiport Switch/1 -> Saturation3/1
  Divide3/1 -> Multiport Switch/3, Multiport Switch/2
  Product4/1 -> [Brake_Trq_out], Brake.Trq.Out/1
  Transfer Fcn LF2/1 -> Product4/1
  [Brake_Trq_in] -> Transfer Fcn LF2/1
  Constant4/1 -> Divide3/2
  [Brake_Trq_in] -> Transfer Fcn LF1/1
  [whl_a] -> Mux/3
  [slipRR] -> RR/7
  [wsd_RR] -> Mux/2
  Mux/1 -> Scope2/1
  [v_whl_switch] -> Mux1/2
  [slipRR] -> Mux1/1
  [v_car_RR] -> RR/1
  [Brake_Trq_in] -> RR/5
  [w_omega_a] -> RR/3
  [Brake_Trq_out] -> RR/6
  [v_car_RR] -> Mux/1
  [phase] -> RR/4
  [wsd_RR] -> RR/2
  Mux1/1 -> Scope6/1
  Read CM Dict2/1 -> RR/8
  Discrete Derivative2/1 -> Gain/1
  [v_car_RR] -> Zero-Order Hold3/1
  Gain/1 -> deceleration_rate/1, [deceleration_rate]
  Switch/1 -> Memory2/1
  Memory2/1 -> Sample and Hold7/Trigger
  Ground/1 -> Switch/3
  [wsd_RR] -> Sample and Hold7/1
  [slipRR] -> Switch/1, Switch/2
  Sample and Hold7/1 -> [v_whl_switch]
  [v_whl_switch] -> Chart_RR/6(v_whl_switch)
  b_trq_min/1 -> Chart_RR/3(b_trq_min)
  [v_car_RR] -> Chart_RR/11(v_car)
  whl_a_max/1 -> Chart_RR/8(whl_a_max)
  [w_omega_a] -> Chart_RR/7(whl_a)
  [slipRR] -> Chart_RR/2(slip)
  [wsd_RR] -> Chart_RR/5(v_whl)
  [Brake_Trq_in] -> Chart_RR/1(b_trq_in)
  whl_a_min/1 -> Chart_RR/9(whl_a_min)
  [slip_switch] -> Chart_RR/4(slip_switch)
  Chart_RR/1(pressure_state) -> Scope/1
  wheelspeed/1 -> [w_omega], wheelspeed [rad/s]/1, Product2/1
  [w_omega] -> Zero-Order Hold2/1
  Saturation3/1 -> Multiport Switch/8, Multiport Switch/6, Multiport Switch/4, Rate Transition4/1, Rate Transition1/1, Rate Transition3/1, Product4/2
  Add1/1 -> Multiport Switch/9
  Add3/1 -> Multiport Switch/5
  Add2/1 -> Multiport Switch/7
  Unit Delay2/1 -> Add2/2
  Unit Delay3/1 -> Add1/2
  Repeating Sequence Stair1/1 -> Add1/1
  Constant3/1 -> Add2/1
  Constant6/1 -> Add3/1
  Unit Delay1/1 -> Add3/2
  Transfer Fcn LF1/1 -> Divide3/1
  Rate Transition4/1 -> Unit Delay1/1
  Rate Transition1/1 -> Unit Delay2/1
  Rate Transition3/1 -> Unit Delay3/1
  Zero-Order Hold1/1 -> Discrete Derivative/1
  Zero-Order Hold2/1 -> Discrete Derivative3/1
  Zero-Order Hold3/1 -> Discrete Derivative2/1
  Discrete Derivative3/1 -> [w_omega_a]
  [deceleration_rate] -> RR/9
  [deceleration_rate] -> Chart_RR/10(deceleration_rate)
  [slipRR] -> Scope_slipRR/1
  Read CM Dict3/1 -> Scope_FxRR/1

== system ABS_virtual_no_fliter_40_88/CarMaker/IPG Vehicle/CarAndTrailer/CarAndTrailerUpd/CreateBus Brake.IF.In ==
  In : Inport
  BusCreator : BusCreator  Inputs=9
  Demux : Demux  Outputs=9
      settings: DisplayOption=none
  Out : Outport  VectorParamsAs1DForOutWhenUnconnected=off
  wires:
  Demux/9 -> BusCreator/9  "Brake IF Trq_Reg RR"
  Demux/8 -> BusCreator/8  "Brake IF Trq_Reg RL"
  Demux/7 -> BusCreator/7  "Brake IF Trq_Reg FR"
  Demux/6 -> BusCreator/6  "Brake IF Trq_Reg FL"
  Demux/5 -> BusCreator/5  "Brake IF Trq_Reg_max RR"
  Demux/4 -> BusCreator/4  "Brake IF Trq_Reg_max RL"
  Demux/3 -> BusCreator/3  "Brake IF Trq_Reg_max FR"
  Demux/2 -> BusCreator/2  "Brake IF Trq_Reg_max FL"
  Demux/1 -> BusCreator/1  "Brake IF T_env"
  BusCreator/1 -> Out/1
  In/1 -> Demux/1

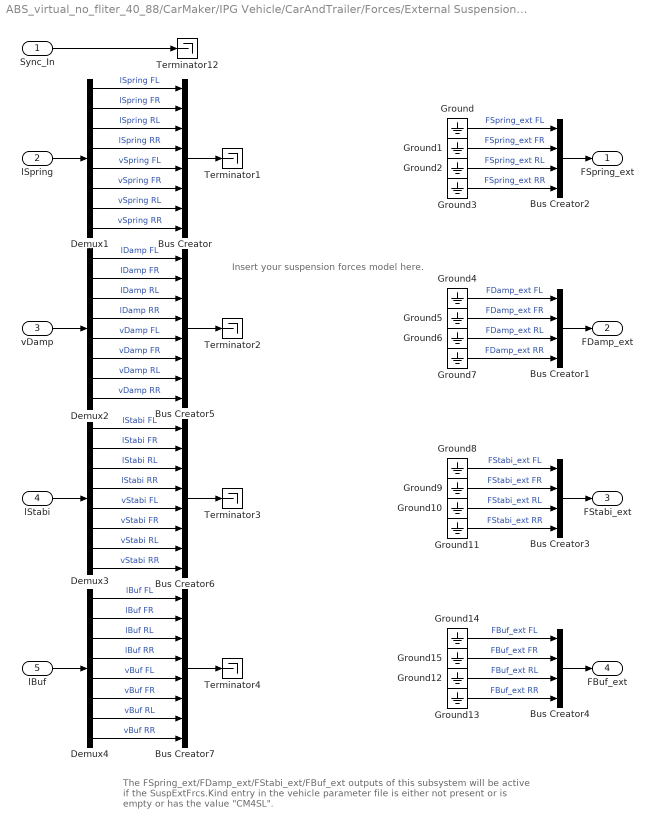
== system ABS_virtual_no_fliter_40_88/CarMaker/IPG Vehicle/CarAndTrailer/Forces/External Suspension Forces ==
  note: The FSpring_ext/FDamp_ext/FStabi_ext/FBuf_ext outputs of this subsystem will be
      | active if the SuspExtFrcs.Kind entry in the vehicle parameter file
      | is either not present or is empty or has the value "CM4SL".
  note: Insert your suspension forces model here.
  Sync_In : Inport
  lSpring : Inport  Port=2
  vDamp : Inport  Port=3
  lStabi : Inport  Port=4
  lBuf : Inport  Port=5
  Bus Creator{,5..7} (4 alike) : BusCreator  Inputs=8
  Bus Creator{1..4} (4 alike) : BusCreator  Inputs=4
  Demux{1..4} (4 alike) : Demux  Outputs=8
      settings: DisplayOption=none
  Ground{,1..15} (16 alike) : Ground
  Terminator{1..4,12} (5 alike) : Terminator
  FSpring_ext : Outport  VectorParamsAs1DForOutWhenUnconnected=off
  FDamp_ext : Outport  Port=2  VectorParamsAs1DForOutWhenUnconnected=off
  FStabi_ext : Outport  Port=3  VectorParamsAs1DForOutWhenUnconnected=off
  FBuf_ext : Outport  Port=4  VectorParamsAs1DForOutWhenUnconnected=off
  wires:
  Bus Creator7/1 -> Terminator4/1
  Bus Creator6/1 -> Terminator3/1
  Bus Creator5/1 -> Terminator2/1
  Bus Creator/1 -> Terminator1/1
  Demux4/8 -> Bus Creator7/8  "vBuf RR"
  Demux4/7 -> Bus Creator7/7  "vBuf RL"
  Demux4/6 -> Bus Creator7/6  "vBuf FR"
  Demux4/5 -> Bus Creator7/5  "vBuf FL"
  Demux3/8 -> Bus Creator6/8  "vStabi RR"
  Demux3/7 -> Bus Creator6/7  "vStabi RL"
  Demux3/6 -> Bus Creator6/6  "vStabi FR"
  Demux3/5 -> Bus Creator6/5  "vStabi FL"
  Demux2/8 -> Bus Creator5/8  "vDamp RR"
  Demux2/7 -> Bus Creator5/7  "vDamp RL"
  Demux2/6 -> Bus Creator5/6  "vDamp FR"
  Demux2/5 -> Bus Creator5/5  "vDamp FL"
  Demux1/8 -> Bus Creator/8  "vSpring RR"
  Demux1/7 -> Bus Creator/7  "vSpring RL"
  Demux1/6 -> Bus Creator/6  "vSpring FR"
  Demux1/5 -> Bus Creator/5  "vSpring FL"
  Demux2/4 -> Bus Creator5/4  "lDamp RR"
  Demux2/3 -> Bus Creator5/3  "lDamp RL"
  Demux2/2 -> Bus Creator5/2  "lDamp FR"
  Demux2/1 -> Bus Creator5/1  "lDamp FL"
  Demux1/4 -> Bus Creator/4  "lSpring RR"
  Demux1/3 -> Bus Creator/3  "lSpring RL"
  Demux1/2 -> Bus Creator/2  "lSpring FR"
  Demux1/1 -> Bus Creator/1  "lSpring FL"
  Demux3/4 -> Bus Creator6/4  "lStabi RR"
  Demux3/3 -> Bus Creator6/3  "lStabi RL"
  Demux3/2 -> Bus Creator6/2  "lStabi FR"
  Demux3/1 -> Bus Creator6/1  "lStabi FL"
  lStabi/1 -> Demux3/1
  vDamp/1 -> Demux2/1
  lSpring/1 -> Demux1/1
  Demux4/4 -> Bus Creator7/4  "lBuf RR"
  Demux4/3 -> Bus Creator7/3  "lBuf RL"
  Demux4/2 -> Bus Creator7/2  "lBuf FR"
  Demux4/1 -> Bus Creator7/1  "lBuf FL"
  lBuf/1 -> Demux4/1
  Ground14/1 -> Bus Creator4/1  "FBuf_ext FL"
  Ground15/1 -> Bus Creator4/2  "FBuf_ext FR"
  Ground12/1 -> Bus Creator4/3  "FBuf_ext RL"
  Ground13/1 -> Bus Creator4/4  "FBuf_ext RR"
  Bus Creator4/1 -> FBuf_ext/1
  Sync_In/1 -> Terminator12/1
  Bus Creator2/1 -> FSpring_ext/1
  Ground/1 -> Bus Creator2/1  "FSpring_ext FL"
  Ground1/1 -> Bus Creator2/2  "FSpring_ext FR"
  Ground2/1 -> Bus Creator2/3  "FSpring_ext RL"
  Ground3/1 -> Bus Creator2/4  "FSpring_ext RR"
  Ground4/1 -> Bus Creator1/1  "FDamp_ext FL"
  Ground5/1 -> Bus Creator1/2  "FDamp_ext FR"
  Ground6/1 -> Bus Creator1/3  "FDamp_ext RL"
  Ground7/1 -> Bus Creator1/4  "FDamp_ext RR"
  Bus Creator1/1 -> FDamp_ext/1
  Ground8/1 -> Bus Creator3/1  "FStabi_ext FL"
  Ground9/1 -> Bus Creator3/2  "FStabi_ext FR"
  Ground10/1 -> Bus Creator3/3  "FStabi_ext RL"
  Ground11/1 -> Bus Creator3/4  "FStabi_ext RR"
  Bus Creator3/1 -> FStabi_ext/1

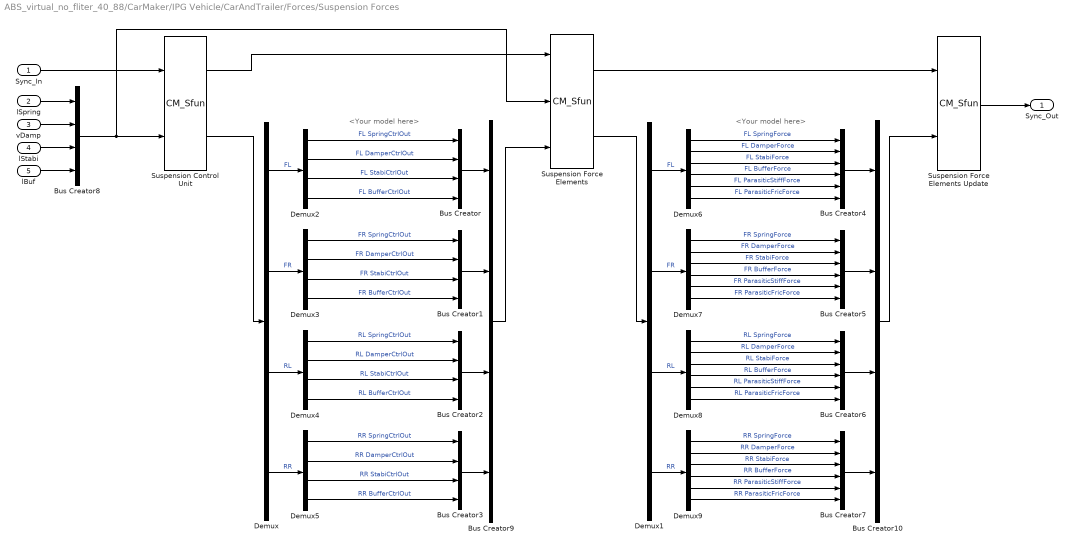
== system ABS_virtual_no_fliter_40_88/CarMaker/IPG Vehicle/CarAndTrailer/Forces/Suspension Forces ==
  note: <Your model here>
  note: <Your model here>
  Sync_In : Inport
  lSpring : Inport  Port=2
  vDamp : Inport  Port=3
  lStabi : Inport  Port=4
  lBuf : Inport  Port=5
  Bus Creator{,1..3,8..10} (7 alike) : BusCreator  Inputs=4
  Bus Creator{4..7} (4 alike) : BusCreator  Inputs=6
  Demux{,1..5} (6 alike) : Demux
  Demux{6..9} (4 alike) : Demux  Outputs=6
  Suspension Control Unit : S-Function  FunctionName=CM_Sfun  Parameters='ForcesSuspControl'  SFunctionDeploymentMode=off  EnableBusSupport=off
  Suspension Force Elements : S-Function  FunctionName=CM_Sfun  Parameters='ForcesSusp'  SFunctionDeploymentMode=off  EnableBusSupport=off
  Suspension Force Elements Update : S-Function  FunctionName=CM_Sfun  Parameters='ForcesSuspUpd'  SFunctionDeploymentMode=off  EnableBusSupport=off
  Sync_Out : Outport  VectorParamsAs1DForOutWhenUnconnected=off
  wires:
  vDamp/1 -> Bus Creator8/2
  lStabi/1 -> Bus Creator8/3
  lBuf/1 -> Bus Creator8/4
  lSpring/1 -> Bus Creator8/1
  Bus Creator8/1 -> Suspension Control Unit/2, Suspension Force Elements/2
  Sync_In/1 -> Suspension Control Unit/1
  Suspension Control Unit/1 -> Suspension Force Elements/1
  Suspension Force Elements/1 -> Suspension Force Elements Update/1
  Suspension Force Elements Update/1 -> Sync_Out/1
  Bus Creator4/1 -> Bus Creator10/1
  Bus Creator5/1 -> Bus Creator10/2
  Bus Creator6/1 -> Bus Creator10/3
  Bus Creator7/1 -> Bus Creator10/4
  Demux6/1 -> Bus Creator4/1  "FL SpringForce"
  Demux9/1 -> Bus Creator7/1  "RR SpringForce"
  Demux9/2 -> Bus Creator7/2  "RR DamperForce"
  Demux9/3 -> Bus Creator7/3  "RR StabiForce"
  Demux9/4 -> Bus Creator7/4  "RR BufferForce"
  Demux9/5 -> Bus Creator7/5  "RR ParasiticStiffForce"
  Demux9/6 -> Bus Creator7/6  "RR ParasiticFricForce"
  Demux8/1 -> Bus Creator6/1  "RL SpringForce"
  Demux8/2 -> Bus Creator6/2  "RL DamperForce"
  Demux8/4 -> Bus Creator6/4  "RL BufferForce"
  Demux8/5 -> Bus Creator6/5  "RL ParasiticStiffForce"
  Demux8/6 -> Bus Creator6/6  "RL ParasiticFricForce"
  Demux8/3 -> Bus Creator6/3  "RL StabiForce"
  Demux7/1 -> Bus Creator5/1  "FR SpringForce"
  Demux7/2 -> Bus Creator5/2  "FR DamperForce"
  Demux7/3 -> Bus Creator5/3  "FR StabiForce"
  Demux7/4 -> Bus Creator5/4  "FR BufferForce"
  Demux7/5 -> Bus Creator5/5  "FR ParasiticStiffForce"
  Demux7/6 -> Bus Creator5/6  "FR ParasiticFricForce"
  Demux6/2 -> Bus Creator4/2  "FL DamperForce"
  Demux6/3 -> Bus Creator4/3  "FL StabiForce"
  Demux6/4 -> Bus Creator4/4  "FL BufferForce"
  Demux6/5 -> Bus Creator4/5  "FL ParasiticStiffForce"
  Demux6/6 -> Bus Creator4/6  "FL ParasiticFricForce"
  Bus Creator10/1 -> Suspension Force Elements Update/2
  Demux/1 -> Demux2/1  "FL"
  Bus Creator1/1 -> Bus Creator9/2
  Demux/2 -> Demux3/1  "FR"
  Bus Creator2/1 -> Bus Creator9/3
  Demux/3 -> Demux4/1  "RL"
  Bus Creator3/1 -> Bus Creator9/4
  Demux2/1 -> Bus Creator/1  "FL SpringCtrlOut"
  Demux/4 -> Demux5/1  "RR"
  Demux5/1 -> Bus Creator3/1  "RR SpringCtrlOut"
  Demux5/2 -> Bus Creator3/2  "RR DamperCtrlOut"
  Demux5/3 -> Bus Creator3/3  "RR StabiCtrlOut"
  Demux5/4 -> Bus Creator3/4  "RR BufferCtrlOut"
  Demux4/1 -> Bus Creator2/1  "RL SpringCtrlOut"
  Demux4/2 -> Bus Creator2/2  "RL DamperCtrlOut"
  Demux4/4 -> Bus Creator2/4  "RL BufferCtrlOut"
  Demux4/3 -> Bus Creator2/3  "RL StabiCtrlOut"
  Demux3/1 -> Bus Creator1/1  "FR SpringCtrlOut"
  Demux3/2 -> Bus Creator1/2  "FR DamperCtrlOut"
  Demux3/3 -> Bus Creator1/3  "FR StabiCtrlOut"
  Demux3/4 -> Bus Creator1/4  "FR BufferCtrlOut"
  Demux2/2 -> Bus Creator/2  "FL DamperCtrlOut"
  Demux2/3 -> Bus Creator/3  "FL StabiCtrlOut"
  Demux2/4 -> Bus Creator/4  "FL BufferCtrlOut"
  Suspension Control Unit/2 -> Demux/1
  Bus Creator9/1 -> Suspension Force Elements/3
  Bus Creator/1 -> Bus Creator9/1
  Suspension Force Elements/2 -> Demux1/1
  Demux1/1 -> Demux6/1  "FL"
  Demux1/2 -> Demux7/1  "FR"
  Demux1/3 -> Demux8/1  "RL"
  Demux1/4 -> Demux9/1  "RR"

== system ABS_virtual_no_fliter_40_88/CarMaker/IPG Vehicle/CarAndTrailer/Forces/Tires ==
  note: The TireXX_Out signals will only be used if FileIdent is "CarMaker-Tire-CM4SL" in the tire parameter file!
      | An example parameter file can be found in Data/Tire/DT_CM4SL_UserTire.
  Sync_In : Inport
  TireFL_In : Inport  Port=2
  TireFR_In : Inport  Port=3
  TireRL_In : Inport  Port=4
  TireRR_In : Inport  Port=5
  Bus Creator{1..4} (4 alike) : BusCreator  Inputs=11
  Demux{1..3,8} (4 alike) : Demux  Outputs=7
      settings: DisplayOption=none
  TireFL : Subsystem
  TireFR : Subsystem
  TireRL : Subsystem
  TireRR : Subsystem
  TireFL_Out : Outport  VectorParamsAs1DForOutWhenUnconnected=off
  TireFR_Out : Outport  Port=2  VectorParamsAs1DForOutWhenUnconnected=off
  TireRL_Out : Outport  Port=3  VectorParamsAs1DForOutWhenUnconnected=off
  TireRR_Out : Outport  Port=4  VectorParamsAs1DForOutWhenUnconnected=off
  wires:
  Sync_In/1 -> TireRR/1(Sync_In), TireRL/1(Sync_In), TireFR/1(Sync_In), TireFL/1(Sync_In)
  Bus Creator4/1 -> TireRR_Out/1
  Bus Creator2/1 -> TireRL_Out/1
  Bus Creator1/1 -> TireFR_Out/1
  Demux3/5 -> TireRR/6(Rim_turnv)  "Tire_In Rim_turnv"
  Demux3/4 -> TireRR/5(Rim_rotv)  "Tire_In Rim_rotv"
  Demux3/1 -> TireRR/2(Load)  "Tire_In Load"
  Demux3/7 -> TireRR/8(muRoad)  "Tire_In mu"
  Demux3/6 -> TireRR/7(InclinAngle)  "Tire_In Camber"
  Demux3/2 -> TireRR/3(vxtrans)  "Tire_In vxtrans"
  Demux3/3 -> TireRR/4(vytrans)  "Tire_In vytrans"
  TireRR/11(AlignTrq) -> Bus Creator4/11  "Tire_Out AlignTrq"
  TireRR/10(RollResist) -> Bus Creator4/10  "Tire_Out RollResist"
  TireRR/9(OverturnTrq) -> Bus Creator4/9  "Tire_Out OverturnTrq"
  TireRR/8(LoadFrc) -> Bus Creator4/8  "Tire_Out LoadFrc"
  TireRR/7(SideFrc) -> Bus Creator4/7  "Tire_Out SideFrc"
  TireRR/6(LongFrc) -> Bus Creator4/6  "Tire_Out LongFrc"
  TireRR/5(vBelt) -> Bus Creator4/5  "Tire_Out vBelt"
  TireRR/4(rBelt_eff) -> Bus Creator4/4  "Tire_Out rBelt_eff"
  TireRR/3(TurnSlp) -> Bus Creator4/3  "Tire_Out TurnSlp"
  TireRR/1(Slp) -> Bus Creator4/1  "Tire_Out Slp"
  TireRR/2(Alpha) -> Bus Creator4/2  "Tire_Out Alpha"
  Demux2/5 -> TireRL/6(Rim_turnv)  "Tire_In Rim_turnv"
  Demux2/4 -> TireRL/5(Rim_rotv)  "Tire_In Rim_rotv"
  Demux2/1 -> TireRL/2(Load)  "Tire_In Load"
  Demux2/7 -> TireRL/8(muRoad)  "Tire_In mu"
  Demux2/6 -> TireRL/7(InclinAngle)  "Tire_In Camber"
  Demux2/2 -> TireRL/3(vxtrans)  "Tire_In vxtrans"
  Demux2/3 -> TireRL/4(vytrans)  "Tire_In vytrans"
  TireRL/11(AlignTrq) -> Bus Creator2/11  "Tire_Out AlignTrq"
  TireRL/10(RollResist) -> Bus Creator2/10  "Tire_Out RollResist"
  TireRL/9(OverturnTrq) -> Bus Creator2/9  "Tire_Out OverturnTrq"
  TireRL/8(LoadFrc) -> Bus Creator2/8  "Tire_Out LoadFrc"
  TireRL/7(SideFrc) -> Bus Creator2/7  "Tire_Out SideFrc"
  TireRL/6(LongFrc) -> Bus Creator2/6  "Tire_Out LongFrc"
  TireRL/5(vBelt) -> Bus Creator2/5  "Tire_Out vBelt"
  TireRL/4(rBelt_eff) -> Bus Creator2/4  "Tire_Out rBelt_eff"
  TireRL/3(TurnSlp) -> Bus Creator2/3  "Tire_Out TurnSlp"
  TireRL/1(Slp) -> Bus Creator2/1  "Tire_Out Slp"
  TireRL/2(Alpha) -> Bus Creator2/2  "Tire_Out Alpha"
  Demux1/5 -> TireFR/6(Rim_turnv)  "Tire_In Rim_turnv"
  Demux1/4 -> TireFR/5(Rim_rotv)  "Tire_In Rim_rotv"
  Demux1/1 -> TireFR/2(Load)  "Tire_In Load"
  Demux1/7 -> TireFR/8(muRoad)  "Tire_In mu"
  Demux1/6 -> TireFR/7(InclinAngle)  "Tire_In Camber"
  Demux1/2 -> TireFR/3(vxtrans)  "Tire_In vxtrans"
  Demux1/3 -> TireFR/4(vytrans)  "Tire_In vytrans"
  TireFR/11(AlignTrq) -> Bus Creator1/11  "Tire_Out AlignTrq"
  TireFR/10(RollResist) -> Bus Creator1/10  "Tire_Out RollResist"
  TireFR/9(OverturnTrq) -> Bus Creator1/9  "Tire_Out OverturnTrq"
  TireFR/8(LoadFrc) -> Bus Creator1/8  "Tire_Out LoadFrc"
  TireFR/7(SideFrc) -> Bus Creator1/7  "Tire_Out SideFrc"
  TireFR/6(LongFrc) -> Bus Creator1/6  "Tire_Out LongFrc"
  TireFR/5(vBelt) -> Bus Creator1/5  "Tire_Out vBelt"
  TireFR/4(rBelt_eff) -> Bus Creator1/4  "Tire_Out rBelt_eff"
  TireFR/3(TurnSlp) -> Bus Creator1/3  "Tire_Out TurnSlp"
  TireFR/1(Slp) -> Bus Creator1/1  "Tire_Out Slp"
  TireFR/2(Alpha) -> Bus Creator1/2  "Tire_Out Alpha"
  Demux8/5 -> TireFL/6(Rim_turnv)  "Tire_In Rim_turnv"
  Demux8/4 -> TireFL/5(Rim_rotv)  "Tire_In Rim_rotv"
  TireFL_In/1 -> Demux8/1
  Demux8/1 -> TireFL/2(Load)  "Tire_In Load"
  Demux8/7 -> TireFL/8(muRoad)  "Tire_In mu"
  Demux8/6 -> TireFL/7(InclinAngle)  "Tire_In Camber"
  Demux8/2 -> TireFL/3(vxtrans)  "Tire_In vxtrans"
  Demux8/3 -> TireFL/4(vytrans)  "Tire_In vytrans"
  TireFL/11(AlignTrq) -> Bus Creator3/11  "Tire_Out AlignTrq"
  TireFL/10(RollResist) -> Bus Creator3/10  "Tire_Out RollResist"
  TireFL/9(OverturnTrq) -> Bus Creator3/9  "Tire_Out OverturnTrq"
  TireFL/8(LoadFrc) -> Bus Creator3/8  "Tire_Out LoadFrc"
  TireFL/7(SideFrc) -> Bus Creator3/7  "Tire_Out SideFrc"
  TireFL/6(LongFrc) -> Bus Creator3/6  "Tire_Out LongFrc"
  TireFL/5(vBelt) -> Bus Creator3/5  "Tire_Out vBelt"
  TireFL/4(rBelt_eff) -> Bus Creator3/4  "Tire_Out rBelt_eff"
  TireFL/3(TurnSlp) -> Bus Creator3/3  "Tire_Out TurnSlp"
  TireFL/1(Slp) -> Bus Creator3/1  "Tire_Out Slp"
  TireFL/2(Alpha) -> Bus Creator3/2  "Tire_Out Alpha"
  Bus Creator3/1 -> TireFL_Out/1
  TireFR_In/1 -> Demux1/1
  TireRL_In/1 -> Demux2/1
  TireRR_In/1 -> Demux3/1

== system ABS_virtual_no_fliter_40_88/CarMaker/IPG Vehicle/CarAndTrailer/Forces/Vehicle Forces ==
  Sync_In : Inport
  Bus Creator1 : BusCreator  Inputs=12
  Bus Creator8 : BusCreator  Inputs=16
  BusCreator1 : BusCreator  Inputs=4
  BusCreator2 : BusCreator  Inputs=9
  Demux : Demux  Outputs=16
      settings: DisplayOption=none
  Demux1 : Demux  Outputs=12
      settings: DisplayOption=none
  Demux2 : Demux  Outputs=13
      settings: DisplayOption=none
  Forces : S-Function  FunctionName=CM_Sfun  Parameters='Forces'  SFunctionDeploymentMode=off  EnableBusSupport=off
  Terminator : Terminator
  Sync_Out : Outport  VectorParamsAs1DForOutWhenUnconnected=off
  Car.Virtual : Outport  Port=2  VectorParamsAs1DForOutWhenUnconnected=off
  Car.Aero : Outport  Port=3  VectorParamsAs1DForOutWhenUnconnected=off
  Car.Load : Outport  Port=4  VectorParamsAs1DForOutWhenUnconnected=off
  wires:
  BusCreator1/1 -> Terminator/1  "Aero IF (in)"
  Demux2/13 -> BusCreator2/9  "car Aero Trq_1 z"
  Demux2/12 -> BusCreator2/8  "car Aero Trq_1 y"
  Demux2/11 -> BusCreator2/7  "car Aero Trq_1 x"
  Demux2/10 -> BusCreator2/6  "car Aero Frc_1 z"
  Demux2/9 -> BusCreator2/5  "car Aero Frc_1 y"
  Demux2/8 -> BusCreator2/4  "car Aero Frc_1 x"
  Demux2/7 -> BusCreator2/3  "car Aero PoA_1 z"
  Demux2/6 -> BusCreator2/2  "car Aero PoA_1 y"
  Demux2/5 -> BusCreator2/1  "car Aero PoA_1 x"
  Demux2/4 -> BusCreator1/4  "car Aero tau_1"
  Demux2/3 -> BusCreator1/3  "car Aero ApproachVel_1 z"
  Demux2/2 -> BusCreator1/2  "car Aero ApproachVel_1 y"
  Demux2/1 -> BusCreator1/1  "car Aero ApproachVel_1 x"
  Demux/16 -> Bus Creator8/16  "Car Load_3 tz"
  Demux/15 -> Bus Creator8/15  "Car Load_3 ty"
  Demux/14 -> Bus Creator8/14  "Car Load_3 tx"
  Demux/13 -> Bus Creator8/13  "Car Load_3 mass"
  Demux1/12 -> Bus Creator1/12  "Car Virtual Trq_0 z"
  Demux1/11 -> Bus Creator1/11  "Car Virtual Trq_0 y"
  Demux1/10 -> Bus Creator1/10  "Car Virtual Trq_0 x"
  Demux1/9 -> Bus Creator1/9  "Car Virtual Trq_1 z"
  Demux1/8 -> Bus Creator1/8  "Car Virtual Trq_1 y"
  Demux1/7 -> Bus Creator1/7  "Car Virtual Trq_1 x"
  Demux1/6 -> Bus Creator1/6  "Car Virtual Frc_0 z"
  Demux1/5 -> Bus Creator1/5  "Car Virtual Frc_0 y"
  Demux1/4 -> Bus Creator1/4  "Car Virtual Frc_0 x"
  Sync_In/1 -> Forces/1
  Forces/1 -> Sync_Out/1
  BusCreator2/1 -> Car.Aero/1
  Demux1/1 -> Bus Creator1/1  "Car Virtual Frc_1 x"
  Demux1/2 -> Bus Creator1/2  "Car Virtual Frc_1 y"
  Demux1/3 -> Bus Creator1/3  "Car Virtual Frc_1 z"
  Forces/3 -> Demux2/1
  Forces/2 -> Demux1/1
  Bus Creator1/1 -> Car.Virtual/1
  Bus Creator8/1 -> Car.Load/1
  Demux/1 -> Bus Creator8/1  "Car Load_0 mass"
  Demux/2 -> Bus Creator8/2  "Car Load_0 tx"
  Demux/3 -> Bus Creator8/3  "Car Load_0 ty"
  Demux/4 -> Bus Creator8/4  "Car Load_0 tz"
  Demux/5 -> Bus Creator8/5  "Car Load_1 mass"
  Demux/6 -> Bus Creator8/6  "Car Load_1 tx"
  Demux/7 -> Bus Creator8/7  "Car Load_1 ty"
  Demux/8 -> Bus Creator8/8  "Car Load_1 tz"
  Demux/9 -> Bus Creator8/9  "Car Load_2 mass"
  Demux/10 -> Bus Creator8/10  "Car Load_2 tx"
  Demux/11 -> Bus Creator8/11  "Car Load_2 ty"
  Demux/12 -> Bus Creator8/12  "Car Load_2 tz"
  Forces/4 -> Demux/1

== system ABS_virtual_no_fliter_40_88/CarMaker/IPG Vehicle/CarAndTrailer/Trailer/CreateBus Car.Hitch.FrcTrq ==
  In1 : Inport
  Bus Creator7 : BusCreator  Inputs=6
  Demux7 : Demux  Outputs=6
      settings: DisplayOption=none
  Out1 : Outport  VectorParamsAs1DForOutWhenUnconnected=off
  wires:
  In1/1 -> Demux7/1
  Bus Creator7/1 -> Out1/1
  Demux7/6 -> Bus Creator7/6  "Car Hitch Trq2Car z"
  Demux7/5 -> Bus Creator7/5  "Car Hitch Trq2Car y"
  Demux7/4 -> Bus Creator7/4  "Car Hitch Trq2Car x"
  Demux7/3 -> Bus Creator7/3  "Car Hitch Frc2Car z"
  Demux7/2 -> Bus Creator7/2  "Car Hitch Frc2Car y"
  Demux7/1 -> Bus Creator7/1  "Car Hitch Frc2Car x"

== system ABS_virtual_no_fliter_40_88/CarMaker/IPG Vehicle/CarAndTrailer/Trailer/CreateBus Vhcl.Motion ==
  In1 : Inport
  BusCreator : BusCreator  Inputs=15
  Demux : Demux  Outputs=15
      settings: DisplayOption=none
  Out1 : Outport  VectorParamsAs1DForOutWhenUnconnected=off
  wires:
  Demux/15 -> BusCreator/15  "Vhcl YawAcc"
  Demux/14 -> BusCreator/14  "Vhcl YawVel"
  Demux/13 -> BusCreator/13  "Vhcl Yaw"
  Demux/12 -> BusCreator/12  "Vhcl PitchAcc"
  Demux/11 -> BusCreator/11  "Vhcl PitchVel"
  Demux/10 -> BusCreator/10  "Vhcl Pitch"
  Demux/9 -> BusCreator/9  "Vhcl RollAcc"
  Demux/8 -> BusCreator/8  "Vhcl RollVel"
  Demux/7 -> BusCreator/7  "Vhcl Roll"
  Demux/6 -> BusCreator/6  "Vhcl Hitch_Pos z"
  Demux/5 -> BusCreator/5  "Vhcl Hitch_Pos y"
  Demux/4 -> BusCreator/4  "Vhcl Hitch_Pos x"
  Demux/3 -> BusCreator/3  "Vhcl sRoad"
  Demux/2 -> BusCreator/2  "Vhcl Distance"
  Demux/1 -> BusCreator/1  "Vhcl v"
  In1/1 -> Demux/1
  BusCreator/1 -> Out1/1

== system ABS_virtual_no_fliter_40_88/CarMaker/IPG Vehicle/CarAndTrailer/Trailer/CreateBus Vhcl.PoI ==
  In1 : Inport
  Bus Creator3 : BusCreator  Inputs=18
  Demux3 : Demux  Outputs=18
      settings: DisplayOption=none
  Out1 : Outport  VectorParamsAs1DForOutWhenUnconnected=off
  wires:
  Demux3/18 -> Bus Creator3/18  "Vhcl PoI_GCS Elev"
  Demux3/17 -> Bus Creator3/17  "Vhcl PoI_GCS Lat"
  Demux3/16 -> Bus Creator3/16  "Vhcl PoI_GCS Long"
  Demux3/15 -> Bus Creator3/15  "Vhcl PoI_Acc_1 z"
  Demux3/14 -> Bus Creator3/14  "Vhcl PoI_Acc_1 y"
  Demux3/13 -> Bus Creator3/13  "Vhcl PoI_Acc_1 x"
  Demux3/12 -> Bus Creator3/12  "Vhcl PoI_Vel_1 z"
  Demux3/11 -> Bus Creator3/11  "Vhcl PoI_Vel_1 y"
  Demux3/10 -> Bus Creator3/10  "Vhcl PoI_Vel_1 x"
  Demux3/9 -> Bus Creator3/9  "Vhcl PoI_Acc z"
  Demux3/8 -> Bus Creator3/8  "Vhcl PoI_Acc y"
  Demux3/7 -> Bus Creator3/7  "Vhcl PoI_Acc x"
  Demux3/6 -> Bus Creator3/6  "Vhcl PoI_Vel z"
  Demux3/5 -> Bus Creator3/5  "Vhcl PoI_Vel y"
  Demux3/4 -> Bus Creator3/4  "Vhcl PoI_Vel x"
  Demux3/3 -> Bus Creator3/3  "Vhcl PoI_Pos z"
  Demux3/2 -> Bus Creator3/2  "Vhcl PoI_Pos y"
  In1/1 -> Demux3/1
  Bus Creator3/1 -> Out1/1
  Demux3/1 -> Bus Creator3/1  "Vhcl PoI_Pos x"
